simulink model "team_division_Dstatic"  (R2023a)
settings: Solver=VariableStepAuto  StartTime=0.0  StopTime=10  RelTol=1e-3
settings Model: Creator=grill  LastModifiedBy=grill

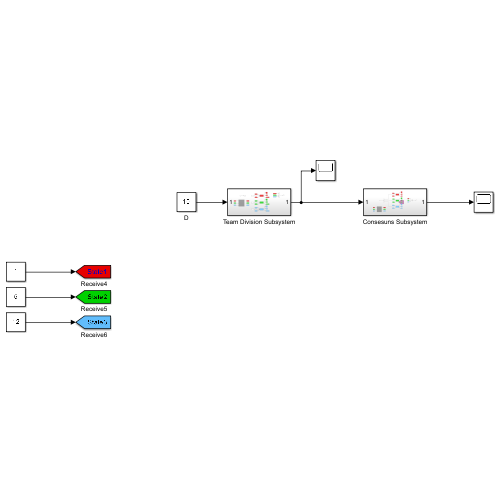
[thumbnail: Simulink's stored preview of the top-level diagram]
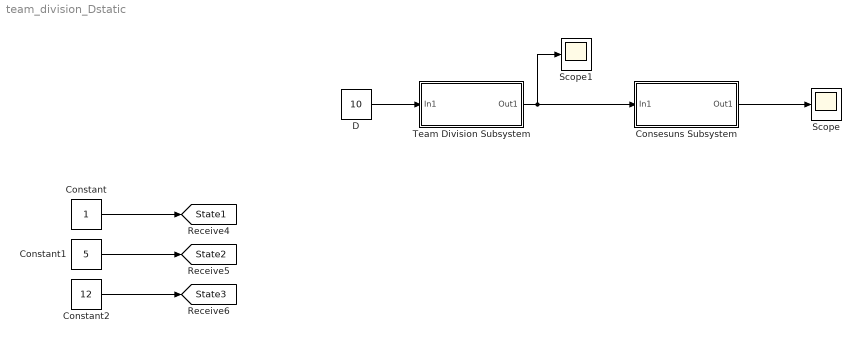
== system team_division_Dstatic ==
  Consesuns Subsystem : Subsystem
  Constant : Constant
  Constant1 : Constant  Value=5
  Constant2 : Constant  Value=12
  D : Constant  Value=10
  Scope : Scope
  Scope1 : Scope
  Team Division Subsystem : Subsystem
  tag scope: State1=global, State2=global, State3=global
  wires:
  D/1 -> Team Division Subsystem/1(In1)
  Consesuns Subsystem/1(Out1) -> Scope/1
  Constant/1 -> [State1]
  Constant1/1 -> [State2]
  Constant2/1 -> [State3]
  Team Division Subsystem/1(Out1) -> Scope1/1, Consesuns Subsystem/1(In1)

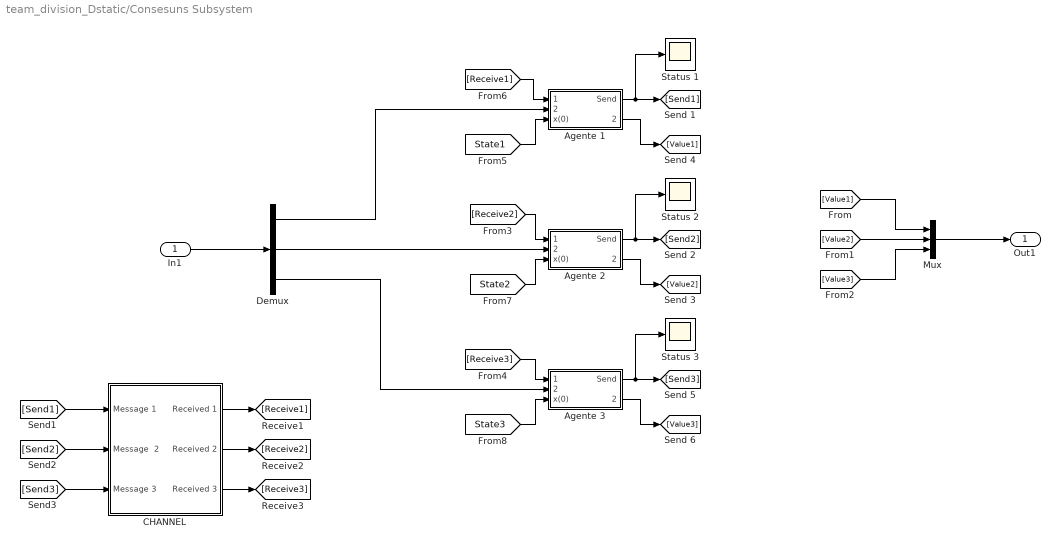
== system team_division_Dstatic/Consesuns Subsystem ==
  In1 : Inport
  Agente 1 : Subsystem
  Agente 2 : Subsystem
  Agente 3 : Subsystem
  CHANNEL : Subsystem
  Demux : Demux  Outputs=3
  Mux : Mux  Inputs=3
  Status 1 : Scope
  Status 2 : Scope
  Status 3 : Scope
  Out1 : Outport
  wires:
  Agente 1/1(Send) -> [Send1], Status 1/1
  In1/1 -> Demux/1
  Mux/1 -> Out1/1
  [Value3] -> Mux/3
  [Value2] -> Mux/2
  [Value1] -> Mux/1
  Demux/1 -> Agente 1/2(team_id)
  Agente 1/2(ValuePort) -> [Value1]
  Agente 2/1(Send) -> [Send2], Status 2/1
  Demux/2 -> Agente 2/2(team_id)
  Agente 2/2(ValuePort) -> [Value2]
  Agente 3/1(Send) -> [Send3], Status 3/1
  Demux/3 -> Agente 3/2(team_id)
  Agente 3/2(ValuePort) -> [Value3]
  [Receive1] -> Agente 1/1(Receive)
  [Receive2] -> Agente 2/1(Receive)
  [Receive3] -> Agente 3/1(Receive)
  [Send1] -> CHANNEL/1(Message 1)
  [Send3] -> CHANNEL/3(Message 3)
  CHANNEL/2(Received 2) -> [Receive2]
  CHANNEL/1(Received 1) -> [Receive1]
  [Send2] -> CHANNEL/2(Message  2)
  CHANNEL/3(Received 3) -> [Receive3]
  [State1] -> Agente 1/3(x(0))
  [State2] -> Agente 2/3(x(0))
  [State3] -> Agente 3/3(x(0))

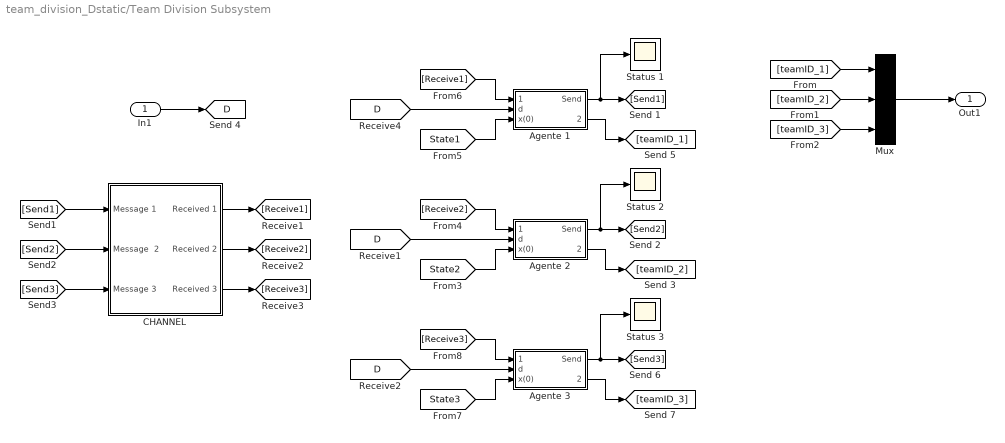
== system team_division_Dstatic/Team Division Subsystem ==
  In1 : Inport
  Agente 1 : Subsystem
  Agente 2 : Subsystem
  Agente 3 : Subsystem
  CHANNEL : Subsystem
  Mux : Mux  Inputs=3
  Status 1 : Scope
  Status 2 : Scope
  Status 3 : Scope
  Out1 : Outport
  tag scope: D=global
  wires:
  Agente 1/1(Send) -> [Send1], Status 1/1
  [D] -> Agente 1/2(d)
  Mux/1 -> Out1/1
  Agente 1/2(TeamPort) -> [teamID_1]
  [teamID_3] -> Mux/3
  [teamID_2] -> Mux/2
  [teamID_1] -> Mux/1
  In1/1 -> [D]
  [Receive1] -> Agente 1/1(Receive)
  [State1] -> Agente 1/3(x(0))
  Agente 2/2(TeamPort) -> [teamID_2]
  [State2] -> Agente 2/3(x(0))
  Agente 2/1(Send) -> [Send2], Status 2/1
  [D] -> Agente 2/2(d)
  [Receive2] -> Agente 2/1(Receive)
  Agente 3/2(TeamPort) -> [teamID_3]
  [State3] -> Agente 3/3(x(0))
  Agente 3/1(Send) -> [Send3], Status 3/1
  [D] -> Agente 3/2(d)
  [Receive3] -> Agente 3/1(Receive)
  CHANNEL/2(Received 2) -> [Receive2]
  [Send1] -> CHANNEL/1(Message 1)
  CHANNEL/1(Received 1) -> [Receive1]
  [Send2] -> CHANNEL/2(Message  2)
  [Send3] -> CHANNEL/3(Message 3)
  CHANNEL/3(Received 3) -> [Receive3]

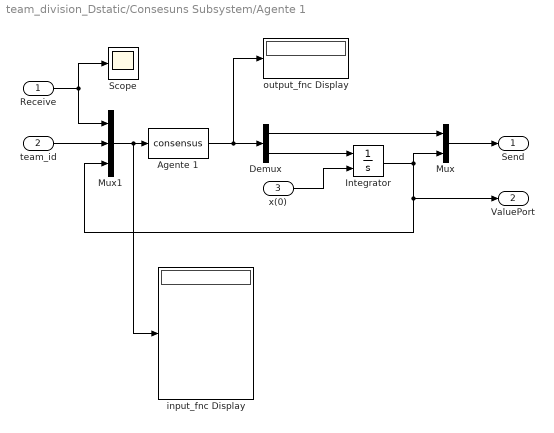
== system team_division_Dstatic/Consesuns Subsystem/Agente 1 ==
  Receive : Inport
  team_id : Inport  Port=2
  x(0) : Inport  Port=3
  Agente 1 : MATLABFcn  MATLABFcn=consensus  OutputDimensions=2
  Demux : Demux  Outputs=2
  Integrator : Integrator  InitialConditionSource=external  InitialCondition=1
  Mux : Mux  Inputs=2
  Mux1 : Mux  Inputs=3
  Scope : Scope
  input_fnc Display : Display
  output_fnc Display : Display
  Send : Outport  VectorParamsAs1DForOutWhenUnconnected=off
  ValuePort : Outport  Port=2
  wires:
  Receive/1 -> Mux1/1, Scope/1
  team_id/1 -> Mux1/2
  Agente 1/1 -> output_fnc Display/1, Demux/1
  Mux/1 -> Send/1
  Demux/1 -> Mux/1
  Mux1/1 -> input_fnc Display/1, Agente 1/1
  Demux/2 -> Integrator/1
  Integrator/1 -> ValuePort/1, Mux1/3, Mux/2
  x(0)/1 -> Integrator/2

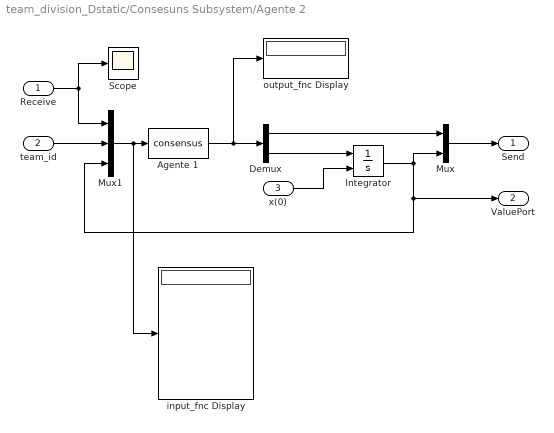
== system team_division_Dstatic/Consesuns Subsystem/Agente 2 ==
  Receive : Inport
  team_id : Inport  Port=2
  x(0) : Inport  Port=3
  Agente 1 : MATLABFcn  MATLABFcn=consensus  OutputDimensions=2
  Demux : Demux  Outputs=2
  Integrator : Integrator  InitialConditionSource=external  InitialCondition=1
  Mux : Mux  Inputs=2
  Mux1 : Mux  Inputs=3
  Scope : Scope
  input_fnc Display : Display
  output_fnc Display : Display
  Send : Outport  VectorParamsAs1DForOutWhenUnconnected=off
  ValuePort : Outport  Port=2
  wires:
  Receive/1 -> Mux1/1, Scope/1
  team_id/1 -> Mux1/2
  Agente 1/1 -> output_fnc Display/1, Demux/1
  Mux/1 -> Send/1
  Demux/1 -> Mux/1
  Mux1/1 -> input_fnc Display/1, Agente 1/1
  Demux/2 -> Integrator/1
  Integrator/1 -> ValuePort/1, Mux1/3, Mux/2
  x(0)/1 -> Integrator/2

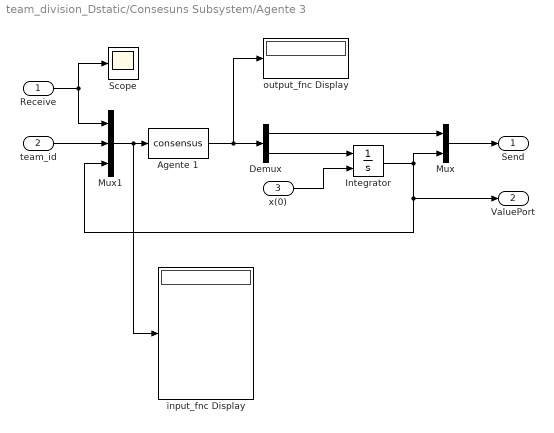
== system team_division_Dstatic/Consesuns Subsystem/Agente 3 ==
  Receive : Inport
  team_id : Inport  Port=2
  x(0) : Inport  Port=3
  Agente 1 : MATLABFcn  MATLABFcn=consensus  OutputDimensions=2
  Demux : Demux  Outputs=2
  Integrator : Integrator  InitialConditionSource=external  InitialCondition=1
  Mux : Mux  Inputs=2
  Mux1 : Mux  Inputs=3
  Scope : Scope
  input_fnc Display : Display
  output_fnc Display : Display
  Send : Outport  VectorParamsAs1DForOutWhenUnconnected=off
  ValuePort : Outport  Port=2
  wires:
  Receive/1 -> Mux1/1, Scope/1
  team_id/1 -> Mux1/2
  Agente 1/1 -> output_fnc Display/1, Demux/1
  Mux/1 -> Send/1
  Demux/1 -> Mux/1
  Mux1/1 -> input_fnc Display/1, Agente 1/1
  Demux/2 -> Integrator/1
  Integrator/1 -> ValuePort/1, Mux1/3, Mux/2
  x(0)/1 -> Integrator/2

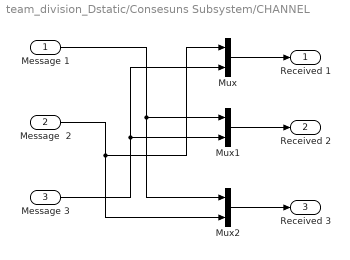
== system team_division_Dstatic/Consesuns Subsystem/CHANNEL ==
  Message 1 : Inport
  Message  2 : Inport  Port=2
  Message 3 : Inport  Port=3
  Mux : Mux  Inputs=2
  Mux1 : Mux  Inputs=2
  Mux2 : Mux  Inputs=2
  Received 1 : Outport  VectorParamsAs1DForOutWhenUnconnected=off
  Received 2 : Outport  Port=2  VectorParamsAs1DForOutWhenUnconnected=off
  Received 3 : Outport  Port=3  VectorParamsAs1DForOutWhenUnconnected=off
  wires:
  Mux2/1 -> Received 3/1
  Mux1/1 -> Received 2/1
  Mux/1 -> Received 1/1
  Message 1/1 -> Mux2/1, Mux1/1
  Message  2/1 -> Mux2/2, Mux/1
  Message 3/1 -> Mux/2, Mux1/2

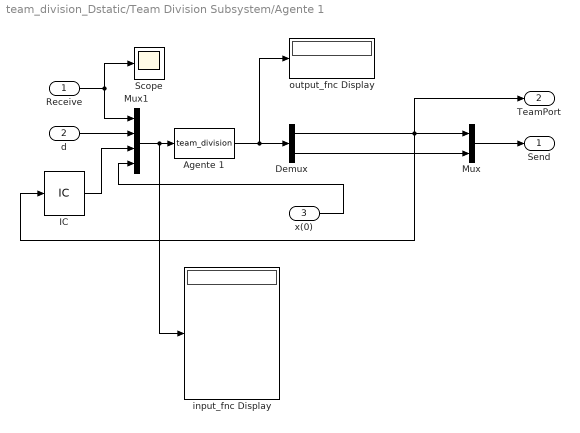
== system team_division_Dstatic/Team Division Subsystem/Agente 1 ==
  Receive : Inport
  d : Inport  Port=2
  x(0) : Inport  Port=3
  Agente 1 : MATLABFcn  MATLABFcn=team_division  OutputDimensions=2
  Demux : Demux  Outputs=2
  IC : InitialCondition  Value=3
  Mux : Mux  Inputs=2
  Mux1 : Mux
  Scope : Scope
  input_fnc Display : Display
  output_fnc Display : Display
  Send : Outport  VectorParamsAs1DForOutWhenUnconnected=off
  TeamPort : Outport  Port=2
  wires:
  Receive/1 -> Mux1/1, Scope/1
  d/1 -> Mux1/2
  IC/1 -> Mux1/3
  Agente 1/1 -> output_fnc Display/1, Demux/1
  Mux/1 -> Send/1
  Demux/1 -> TeamPort/1, Mux/1, IC/1
  Mux1/1 -> input_fnc Display/1, Agente 1/1
  Demux/2 -> Mux/2
  x(0)/1 -> Mux1/4

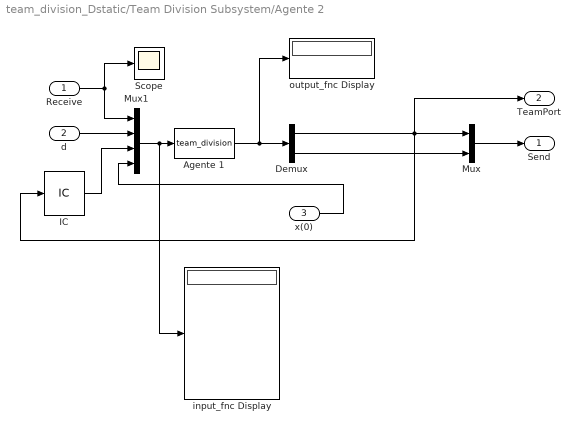
== system team_division_Dstatic/Team Division Subsystem/Agente 2 ==
  Receive : Inport
  d : Inport  Port=2
  x(0) : Inport  Port=3
  Agente 1 : MATLABFcn  MATLABFcn=team_division  OutputDimensions=2
  Demux : Demux  Outputs=2
  IC : InitialCondition  Value=6
  Mux : Mux  Inputs=2
  Mux1 : Mux
  Scope : Scope
  input_fnc Display : Display
  output_fnc Display : Display
  Send : Outport  VectorParamsAs1DForOutWhenUnconnected=off
  TeamPort : Outport  Port=2
  wires:
  Receive/1 -> Mux1/1, Scope/1
  d/1 -> Mux1/2
  IC/1 -> Mux1/3
  Agente 1/1 -> output_fnc Display/1, Demux/1
  Mux/1 -> Send/1
  Demux/1 -> TeamPort/1, Mux/1, IC/1
  Mux1/1 -> input_fnc Display/1, Agente 1/1
  Demux/2 -> Mux/2
  x(0)/1 -> Mux1/4

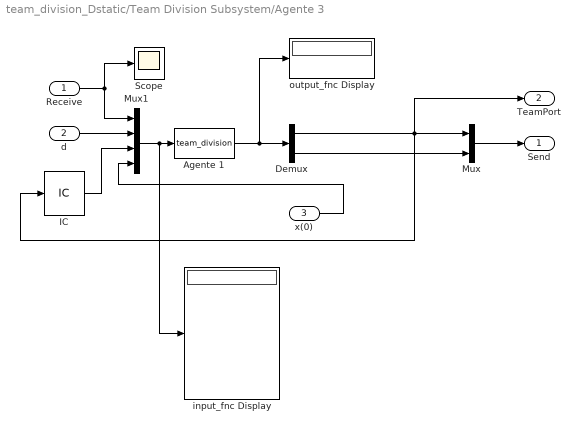
== system team_division_Dstatic/Team Division Subsystem/Agente 3 ==
  Receive : Inport
  d : Inport  Port=2
  x(0) : Inport  Port=3
  Agente 1 : MATLABFcn  MATLABFcn=team_division  OutputDimensions=2
  Demux : Demux  Outputs=2
  IC : InitialCondition  Value=12
  Mux : Mux  Inputs=2
  Mux1 : Mux
  Scope : Scope
  input_fnc Display : Display
  output_fnc Display : Display
  Send : Outport  VectorParamsAs1DForOutWhenUnconnected=off
  TeamPort : Outport  Port=2
  wires:
  Receive/1 -> Mux1/1, Scope/1
  d/1 -> Mux1/2
  IC/1 -> Mux1/3
  Agente 1/1 -> output_fnc Display/1, Demux/1
  Mux/1 -> Send/1
  Demux/1 -> TeamPort/1, Mux/1, IC/1
  Mux1/1 -> input_fnc Display/1, Agente 1/1
  Demux/2 -> Mux/2
  x(0)/1 -> Mux1/4

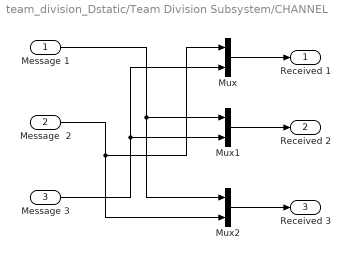
== system team_division_Dstatic/Team Division Subsystem/CHANNEL ==
  Message 1 : Inport
  Message  2 : Inport  Port=2
  Message 3 : Inport  Port=3
  Mux : Mux  Inputs=2
  Mux1 : Mux  Inputs=2
  Mux2 : Mux  Inputs=2
  Received 1 : Outport  VectorParamsAs1DForOutWhenUnconnected=off
  Received 2 : Outport  Port=2  VectorParamsAs1DForOutWhenUnconnected=off
  Received 3 : Outport  Port=3  VectorParamsAs1DForOutWhenUnconnected=off
  wires:
  Mux2/1 -> Received 3/1
  Mux1/1 -> Received 2/1
  Mux/1 -> Received 1/1
  Message 1/1 -> Mux2/1, Mux1/1
  Message  2/1 -> Mux2/2, Mux/1
  Message 3/1 -> Mux/2, Mux1/2
